simulink model "udpTest"  (R2024a)
settings: Solver=VariableStepAuto  StartTime=0.0  StopTime=10.0  RelTol=1e-3
undefined symbols (not defined in the file): f
libraries: instrumentlib x2, dspnetwork x1
settings Model: Creator=nate  LastModifiedBy=nate

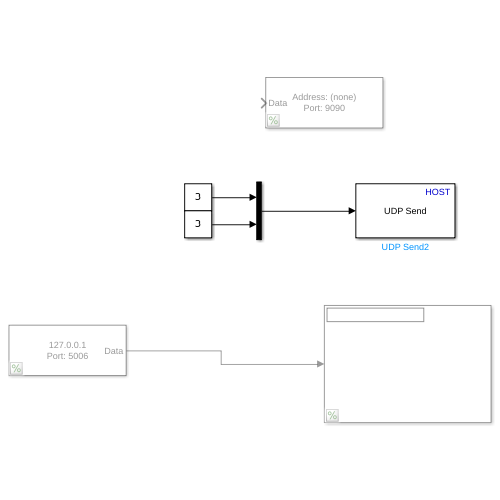
[thumbnail: Simulink's stored preview of the top-level diagram]
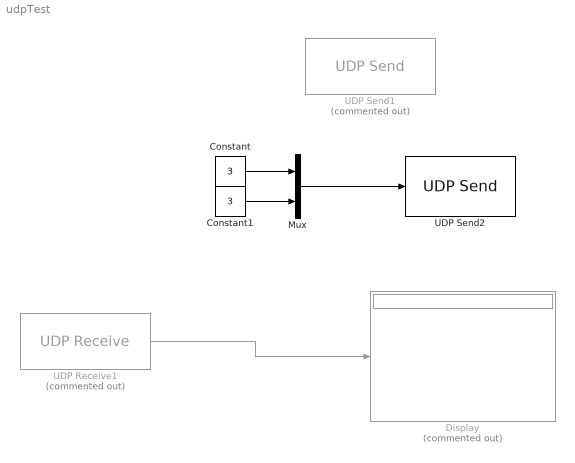
== system udpTest ==
  Constant : Constant  Value=3
  Constant1 : Constant  Value=3
  Display : Display  Commented=on
  Mux : Mux  Inputs=2
  UDP Receive1 : instrumentlib/UDP Receive  Commented=on  LocalAddress=127.0.0.1  LocalPort=5006  EnablePortSharing=off  Host=localhost  Port=9090  GetLatestData=off  DataSize=[ 1, 4]  DataType=uint8  ASCIIFormatting=%f,  Terminator=LF  CustomTerminator=10  ByteOrder=big-endian  EnableBlockingMode=on  Timeout=10  SampleTime=0.01  SimulateUsing=Interpreted execution
  UDP Send1 : instrumentlib/UDP Send  Commented=on  Port=9090  LocalAddress=0.0.0.0  LocalPort=-1  EnablePortSharing=off  OutputDatagramPacketSize=512  ByteOrder=big-endian  EnableBlockingMode=on  SimulateUsing=Interpreted execution
  UDP Send2 : dspnetwork/UDP Send  remoteURL='127.0.0.1'  remotePort=5005  localURL='0.0.0.0'  localPortSource=Automatically determine  localPort=-1  sendBufferSize=1024  sampletime=-1  blockPlatform=HOST  separateLengthPort=0
      settings: LibrarySourceBlock=embeddedtargetslib/Host Communication/UDP Send
  wires:
  UDP Receive1/1 -> Display/1
  Constant/1 -> Mux/1
  Constant1/1 -> Mux/2
  Mux/1 -> UDP Send2/1
